simulink model "delay_bram_prog_blk"  (R2019a)
settings: Solver=VariableStepAuto  StartTime=0.0  StopTime=20  RelTol=1e-3
libraries: xbsIndex_r4 x1
settings Model: Creator=mybur  LastModifiedBy=mybur

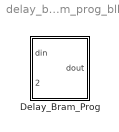
== system delay_bram_prog_blk ==
  Delay_Bram_Prog : Subsystem  mask{max_delay=5, ram_latency=3, bram_primitive="block"}
      mask prompts: max_delay "Max Delay (2^?)"; ram_latency "BRAM Latency"; bram_primitive "BRAM Primitive"
      mask init:
      | Simulink.Block.eval([gcb, '/delay_bram_prog']);
      mask TypeOptions bram_primitive: "block" | "distributed" | "auto" | "ultra"

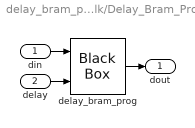
== system delay_bram_prog_blk/Delay_Bram_Prog ==
  din : Inport
  delay : Inport  Port=2
  delay_bram_prog : xbsIndex_r4/Black Box  init_code=delay_bram_prog_config  sim_method=ISE Simulator  verbose=off  block_type=blackbox2
  dout : Outport
  wires:
  din/1 -> delay_bram_prog/1
  delay_bram_prog/1 -> dout/1
  delay/1 -> delay_bram_prog/2
